simulink model "pcssp_PID_sensor"  (R2021b)
settings: Solver=VariableStepAuto  StartTime=0.0  StopTime=10.0  RelTol=1e-3
undefined symbols (not defined in the file or in its folder): pcssp_PID_sensor_fp
settings Model: DataDictionary=pcssp_PID_sensor.sldd  Creator=ravenst1  LastModifiedBy=timoravensbergen
settings SolverCC: AlgebraicLoopSolver=TrustRegion

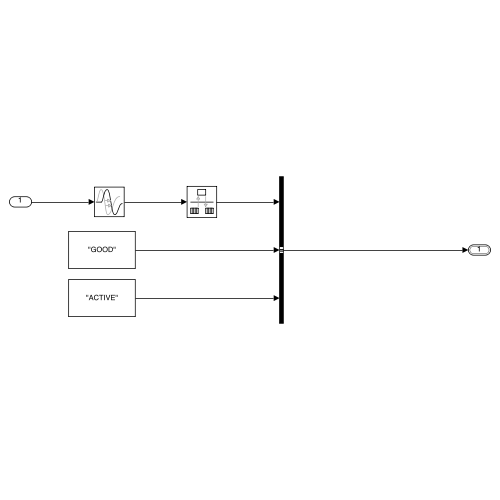
[thumbnail: Simulink's stored preview of the top-level diagram]
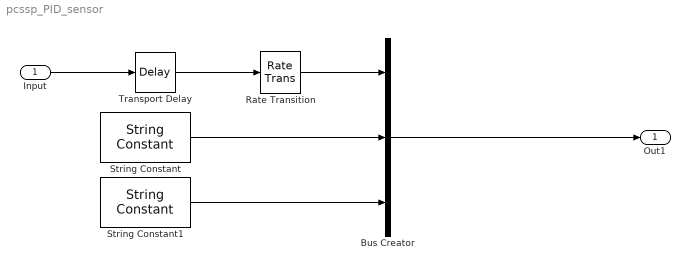
== system pcssp_PID_sensor ==
  Input : Inport
  Bus Creator : BusCreator  Inputs=3  OutDataTypeStr=Bus: PcsSignal
      settings: InheritFromInputs=off
  Rate Transition : RateTransition
  String Constant : StringConstant  String="\"GOOD\""
  String Constant1 : StringConstant  String="\"ACTIVE\""
  Transport Delay : TransportDelay  DelayTime=pcssp_PID_sensor_fp.delay
  Out1 : Outport  OutDataTypeStr=Bus: PcsSignal
  wires:
  Input/1 -> Transport Delay/1
  Bus Creator/1 -> Out1/1
  Transport Delay/1 -> Rate Transition/1
  String Constant/1 -> Bus Creator/2
  String Constant1/1 -> Bus Creator/3
  Rate Transition/1 -> Bus Creator/1
